simulink model "MC_Phase2_Part1_Q2_Sim"  (R2018b)
settings: Solver=VariableStepAuto  StartTime=0.0  StopTime=20.0  RelTol=1e-3
settings Model: Creator=ASUS  LastModifiedBy=1007
settings DataIOCC: ReturnWorkspaceOutputs=on

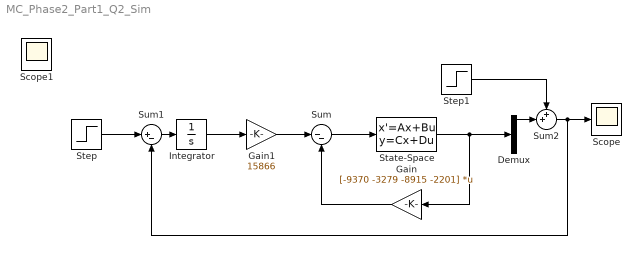
== system MC_Phase2_Part1_Q2_Sim ==
  Demux : Demux
  Gain : Gain  Gain=[-9370 -3279 -8915 -2201]  Multiplication=Matrix(K*u)
  Gain1 : Gain  Gain=15866
  Integrator : Integrator
  Scope : Scope
  State-Space : StateSpace  A=[0 1 0 0;0 -2.2626 -0.3963 0.0082;0 0 0 1;0 3.5649 16.0655 -0.3324]  B=[0;0.2263;0;-0.3565]  C=[1 0 0 0;0 1 0 0;0 0 1 0;0 0 0 1]  D=[0;0;0;0]  InitialCondition=0
  Step : Step  SampleTime=0
  Step1 : Step  Time=5  After=0.3  SampleTime=0
  Sum : Sum  Inputs=|--
  Sum1 : Sum  Inputs=|+-
  Sum2 : Sum  Inputs=++|
  Scope1 : Scope
  wires:
  State-Space/1 -> Gain/1, Demux/1
  Gain/1 -> Sum/2
  Sum/1 -> State-Space/1
  Step/1 -> Sum1/1
  Sum1/1 -> Integrator/1
  Gain1/1 -> Sum/1
  Integrator/1 -> Gain1/1
  Sum2/1 -> Sum1/2, Scope/1
  Demux/1 -> Sum2/2
  Step1/1 -> Sum2/1
